simulink model "model_sym"  (R2018a)
settings: Solver=VariableStepAuto  StartTime=0.0  StopTime=10.0  RelTol=1e-3
libraries: simulink x4
settings Model: PauseTimes=20  Creator=Nikita  LastModifiedBy=Nikita

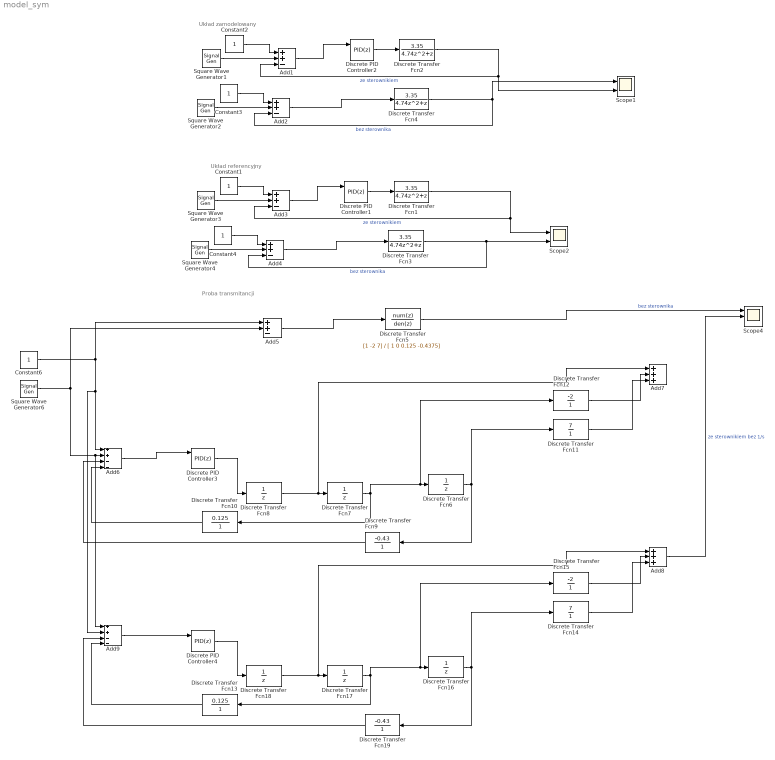
== system model_sym ==
  note: Układ zamodelowany
  note: Układ referencyjny
  note: Proba transmitancji
  Add{1..5} (5 alike) : Sum  Inputs=++-
  Add6 : Sum  Inputs=++--
  Add7 : Sum  Inputs=+++
  Add8 : Sum  Inputs=+++
  Add9 : Sum  Inputs=++--
  Constant{1..4,6} (5 alike) : Constant
  Discrete Transfer Fcn{1..4} (4 alike) : DiscreteTransferFcn  Numerator=[3.35]  Denominator=[ 4.74 1 0]  SampleTime=0.005
  Discrete Transfer Fcn10 : DiscreteTransferFcn  Numerator=[0.125]  Denominator=[ 1 ]  SampleTime=0.005
  Discrete Transfer Fcn11 : DiscreteTransferFcn  Numerator=[7]  Denominator=[1]  SampleTime=0.005
  Discrete Transfer Fcn12 : DiscreteTransferFcn  Numerator=[-2]  Denominator=[1]  SampleTime=0.005
  Discrete Transfer Fcn13 : DiscreteTransferFcn  Numerator=[0.125]  Denominator=[ 1 ]  SampleTime=0.005
  Discrete Transfer Fcn14 : DiscreteTransferFcn  Numerator=[7]  Denominator=[1]  SampleTime=0.005
  Discrete Transfer Fcn15 : DiscreteTransferFcn  Numerator=[-2]  Denominator=[1]  SampleTime=0.005
  Discrete Transfer Fcn{6..8,16..18} (6 alike) : DiscreteTransferFcn  Denominator=[ 1 0 ]  SampleTime=0.005
  Discrete Transfer Fcn19 : DiscreteTransferFcn  Numerator=[-0.43]  Denominator=[1]  SampleTime=0.005
  Discrete Transfer Fcn5 : DiscreteTransferFcn  Numerator=[1 -2 7]  Denominator=[ 1 0 0.125 -0.4375]  SampleTime=0.005
  Discrete Transfer Fcn9 : DiscreteTransferFcn  Numerator=[-0.43]  Denominator=[1]  SampleTime=0.005
  Discrete PID Controller1 : simulink/Continuous/PID Controller  Controller=PID  TimeDomain=Discrete-time  SampleTime=-1  IntegratorMethod=Forward Euler  FilterMethod=Forward Euler  Form=Parallel  UseFilter=on  ControllerParametersSource=internal  P=0.468872547138011  I=87.2715429291033  D=-0.00380212754886475  N=56.6045414469178  InitialConditionSource=internal  InitialConditionForIntegrator=0  InitialConditionForFilter=0  ExternalReset=level  LimitOutput=off  UpperSaturationLimit=inf  LowerSaturationLimit=-inf  LinearizeAsGain=off  AntiWindupMode=none  Kb=1  TrackingMode=off  Kt=1  PParamMin=[]  PParamMax=[]  IParamMin=[]  IParamMax=[]  DParamMin=[]  DParamMax=[]  NParamMin=[]  NParamMax=[]  KbParamMin=[]  KbParamMax=[]  KtParamMin=[]  KtParamMax=[]  POutMin=[]  POutMax=[]  IOutMin=[]  IOutMax=[]  DOutMin=[]  DOutMax=[]  NOutMin=[]  NOutMax=[]  KbOutMin=[]  KbOutMax=[]  KtOutMin=[]  KtOutMax=[]  IntegratorOutMin=[]  IntegratorOutMax=[]  FilterOutMin=[]  FilterOutMax=[]  SumOutMin=[]  SumOutMax=[]  SumI1OutMin=[]  SumI1OutMax=[]  SumI2OutMin=[]  SumI2OutMax=[]  SumI3OutMin=[]  SumI3OutMax=[]  SumDOutMin=[]  SumDOutMax=[]  SaturationOutMin=[]  SaturationOutMax=[]  IntegratorContinuousStateAttributes=''  IntegratorStateMustResolveToSignalObject=off  IntegratorRTWStateStorageClass=Auto  FilterContinuousStateAttributes=''  FilterStateMustResolveToSignalObject=off  FilterRTWStateStorageClass=Auto  DifferentiatorICPrevScaledInput=0  DifferentiatorOutMin=[]  DifferentiatorOutMax=[]  FilterDiffOutCoefMin=[]  FilterDiffOutCoefMax=[]  SumDenOutMin=[]  SumDenOutMax=[]  SumNumOutMin=[]  SumNumOutMax=[]  ReciprocalOutMin=[]  ReciprocalOutMax=[]  DivideOutMin=[]  DivideOutMax=[]  TunerSelectOption=Transfer Function Based (PID Tuner App)
  Discrete PID Controller2 : simulink/Continuous/PID Controller  Controller=PID  TimeDomain=Discrete-time  SampleTime=-1  IntegratorMethod=Forward Euler  FilterMethod=Forward Euler  Form=Parallel  UseFilter=on  ControllerParametersSource=internal  P=0.468872547138011  I=87.2715429291033  D=-0.00380212754886475  N=56.6045414469178  InitialConditionSource=internal  InitialConditionForIntegrator=0  InitialConditionForFilter=0  ExternalReset=level  LimitOutput=off  UpperSaturationLimit=inf  LowerSaturationLimit=-inf  LinearizeAsGain=off  AntiWindupMode=none  Kb=1  TrackingMode=off  Kt=1  PParamMin=[]  PParamMax=[]  IParamMin=[]  IParamMax=[]  DParamMin=[]  DParamMax=[]  NParamMin=[]  NParamMax=[]  KbParamMin=[]  KbParamMax=[]  KtParamMin=[]  KtParamMax=[]  POutMin=[]  POutMax=[]  IOutMin=[]  IOutMax=[]  DOutMin=[]  DOutMax=[]  NOutMin=[]  NOutMax=[]  KbOutMin=[]  KbOutMax=[]  KtOutMin=[]  KtOutMax=[]  IntegratorOutMin=[]  IntegratorOutMax=[]  FilterOutMin=[]  FilterOutMax=[]  SumOutMin=[]  SumOutMax=[]  SumI1OutMin=[]  SumI1OutMax=[]  SumI2OutMin=[]  SumI2OutMax=[]  SumI3OutMin=[]  SumI3OutMax=[]  SumDOutMin=[]  SumDOutMax=[]  SaturationOutMin=[]  SaturationOutMax=[]  IntegratorContinuousStateAttributes=''  IntegratorStateMustResolveToSignalObject=off  IntegratorRTWStateStorageClass=Auto  FilterContinuousStateAttributes=''  FilterStateMustResolveToSignalObject=off  FilterRTWStateStorageClass=Auto  DifferentiatorICPrevScaledInput=0  DifferentiatorOutMin=[]  DifferentiatorOutMax=[]  FilterDiffOutCoefMin=[]  FilterDiffOutCoefMax=[]  SumDenOutMin=[]  SumDenOutMax=[]  SumNumOutMin=[]  SumNumOutMax=[]  ReciprocalOutMin=[]  ReciprocalOutMax=[]  DivideOutMin=[]  DivideOutMax=[]  TunerSelectOption=Transfer Function Based (PID Tuner App)
  Discrete PID Controller3 : simulink/Continuous/PID Controller  Controller=PID  TimeDomain=Discrete-time  SampleTime=-1  IntegratorMethod=Forward Euler  FilterMethod=Forward Euler  Form=Parallel  UseFilter=on  ControllerParametersSource=internal  P=0.468872547138011  I=87.2715429291033  D=-0.00380212754886475  N=56.6045414469178  InitialConditionSource=internal  InitialConditionForIntegrator=0  InitialConditionForFilter=0  ExternalReset=level  LimitOutput=off  UpperSaturationLimit=inf  LowerSaturationLimit=-inf  LinearizeAsGain=off  AntiWindupMode=none  Kb=1  TrackingMode=off  Kt=1  PParamMin=[]  PParamMax=[]  IParamMin=[]  IParamMax=[]  DParamMin=[]  DParamMax=[]  NParamMin=[]  NParamMax=[]  KbParamMin=[]  KbParamMax=[]  KtParamMin=[]  KtParamMax=[]  POutMin=[]  POutMax=[]  IOutMin=[]  IOutMax=[]  DOutMin=[]  DOutMax=[]  NOutMin=[]  NOutMax=[]  KbOutMin=[]  KbOutMax=[]  KtOutMin=[]  KtOutMax=[]  IntegratorOutMin=[]  IntegratorOutMax=[]  FilterOutMin=[]  FilterOutMax=[]  SumOutMin=[]  SumOutMax=[]  SumI1OutMin=[]  SumI1OutMax=[]  SumI2OutMin=[]  SumI2OutMax=[]  SumI3OutMin=[]  SumI3OutMax=[]  SumDOutMin=[]  SumDOutMax=[]  SaturationOutMin=[]  SaturationOutMax=[]  IntegratorContinuousStateAttributes=''  IntegratorStateMustResolveToSignalObject=off  IntegratorRTWStateStorageClass=Auto  FilterContinuousStateAttributes=''  FilterStateMustResolveToSignalObject=off  FilterRTWStateStorageClass=Auto  DifferentiatorICPrevScaledInput=0  DifferentiatorOutMin=[]  DifferentiatorOutMax=[]  FilterDiffOutCoefMin=[]  FilterDiffOutCoefMax=[]  SumDenOutMin=[]  SumDenOutMax=[]  SumNumOutMin=[]  SumNumOutMax=[]  ReciprocalOutMin=[]  ReciprocalOutMax=[]  DivideOutMin=[]  DivideOutMax=[]  TunerSelectOption=Transfer Function Based (PID Tuner App)
  Discrete PID Controller4 : simulink/Continuous/PID Controller  Controller=PID  TimeDomain=Discrete-time  SampleTime=-1  IntegratorMethod=Forward Euler  FilterMethod=Forward Euler  Form=Parallel  UseFilter=on  ControllerParametersSource=internal  P=0.468872547138011  I=0  D=-0.00380212754886475  N=56.6045414469178  InitialConditionSource=internal  InitialConditionForIntegrator=0  InitialConditionForFilter=0  ExternalReset=level  LimitOutput=off  UpperSaturationLimit=inf  LowerSaturationLimit=-inf  LinearizeAsGain=off  AntiWindupMode=none  Kb=1  TrackingMode=off  Kt=1  PParamMin=[]  PParamMax=[]  IParamMin=[]  IParamMax=[]  DParamMin=[]  DParamMax=[]  NParamMin=[]  NParamMax=[]  KbParamMin=[]  KbParamMax=[]  KtParamMin=[]  KtParamMax=[]  POutMin=[]  POutMax=[]  IOutMin=[]  IOutMax=[]  DOutMin=[]  DOutMax=[]  NOutMin=[]  NOutMax=[]  KbOutMin=[]  KbOutMax=[]  KtOutMin=[]  KtOutMax=[]  IntegratorOutMin=[]  IntegratorOutMax=[]  FilterOutMin=[]  FilterOutMax=[]  SumOutMin=[]  SumOutMax=[]  SumI1OutMin=[]  SumI1OutMax=[]  SumI2OutMin=[]  SumI2OutMax=[]  SumI3OutMin=[]  SumI3OutMax=[]  SumDOutMin=[]  SumDOutMax=[]  SaturationOutMin=[]  SaturationOutMax=[]  IntegratorContinuousStateAttributes=''  IntegratorStateMustResolveToSignalObject=off  IntegratorRTWStateStorageClass=Auto  FilterContinuousStateAttributes=''  FilterStateMustResolveToSignalObject=off  FilterRTWStateStorageClass=Auto  DifferentiatorICPrevScaledInput=0  DifferentiatorOutMin=[]  DifferentiatorOutMax=[]  FilterDiffOutCoefMin=[]  FilterDiffOutCoefMax=[]  SumDenOutMin=[]  SumDenOutMax=[]  SumNumOutMin=[]  SumNumOutMax=[]  ReciprocalOutMin=[]  ReciprocalOutMax=[]  DivideOutMin=[]  DivideOutMax=[]  TunerSelectOption=Transfer Function Based (PID Tuner App)
  Scope1 : Scope  NumInputPorts=2
  Scope2 : Scope  NumInputPorts=2
  Scope4 : Scope  NumInputPorts=3
  Square Wave Generator{1..4} (4 alike) : SignalGenerator  WaveForm=square  Frequency=10  Units=rad/sec
  Square Wave Generator6 : SignalGenerator  WaveForm=square  Units=rad/sec
  wires:
  Add1/1 -> Discrete PID Controller2/1
  Square Wave Generator1/1 -> Add1/2
  Discrete PID Controller2/1 -> Discrete Transfer Fcn2/1
  Constant2/1 -> Add1/1
  Discrete Transfer Fcn2/1 -> Scope1/2, Add1/3  "ze sterownikiem"
  Discrete Transfer Fcn4/1 -> Scope1/1, Add2/3  "bez sterownika"
  Constant3/1 -> Add2/1
  Add2/1 -> Discrete Transfer Fcn4/1
  Square Wave Generator2/1 -> Add2/2
  Square Wave Generator4/1 -> Add4/2
  Add4/1 -> Discrete Transfer Fcn3/1
  Constant4/1 -> Add4/1
  Discrete Transfer Fcn3/1 -> Scope2/2, Add4/3  "bez sterownika"
  Discrete Transfer Fcn1/1 -> Scope2/1, Add3/3  "ze sterownikiem"
  Constant1/1 -> Add3/1
  Discrete PID Controller1/1 -> Discrete Transfer Fcn1/1
  Square Wave Generator3/1 -> Add3/2
  Add3/1 -> Discrete PID Controller1/1
  Square Wave Generator6/1 -> Add5/2, Add9/1, Add6/2
  Constant6/1 -> Add6/1, Add9/2, Add5/1
  Add5/1 -> Discrete Transfer Fcn5/1
  Discrete Transfer Fcn7/1 -> Discrete Transfer Fcn12/1, Discrete Transfer Fcn6/1, Discrete Transfer Fcn10/1
  Discrete Transfer Fcn10/1 -> Add6/4
  Discrete Transfer Fcn6/1 -> Discrete Transfer Fcn9/1, Discrete Transfer Fcn11/1
  Discrete Transfer Fcn9/1 -> Add6/3
  Discrete Transfer Fcn8/1 -> Add7/1, Discrete Transfer Fcn7/1
  Discrete Transfer Fcn12/1 -> Add7/2
  Discrete Transfer Fcn11/1 -> Add7/3
  Discrete Transfer Fcn5/1 -> Scope4/1  "bez sterownika"
  Add6/1 -> Discrete PID Controller3/1
  Discrete PID Controller3/1 -> Discrete Transfer Fcn8/1
  Discrete PID Controller4/1 -> Discrete Transfer Fcn18/1
  Discrete Transfer Fcn14/1 -> Add8/3
  Discrete Transfer Fcn15/1 -> Add8/2
  Discrete Transfer Fcn18/1 -> Discrete Transfer Fcn17/1, Add8/1
  Discrete Transfer Fcn19/1 -> Add9/3
  Discrete Transfer Fcn16/1 -> Discrete Transfer Fcn14/1, Discrete Transfer Fcn19/1
  Discrete Transfer Fcn13/1 -> Add9/4
  Discrete Transfer Fcn17/1 -> Discrete Transfer Fcn13/1, Discrete Transfer Fcn16/1, Discrete Transfer Fcn15/1
  Add9/1 -> Discrete PID Controller4/1
  Add8/1 -> Scope4/2  "ze sterownikiem bez 1/s"
